simulink model "rev_3f_UW"  (Simulink 8.4)
settings: Solver=ode23tb  StartTime=0.0  StopTime=0.3  MaxStep=2e-4  RelTol=1e-3  AbsTol=1e-6
libraries: powerlib x22, powerlib_extras x6
settings Model: Creator=Teacher  LastModifiedBy=Student
settings SolverCC: ZeroCrossAlgorithm=Adaptive
settings DataIOCC: LimitDataPoints=off  SaveOutput=off  SaveTime=off
settings OptimizationCC: BlockReduction=off  BooleanDataType=off  ExpressionDepthLimit=128  InitFltsAndDblsToZero=on
settings DebuggingCC: SaveWithParameterizedLinksMsg=none  SignalResolutionControl=TryResolveAllWithWarning  SolverPrmCheckMsg=none  MultiTaskDSMMsg=warning  MultiTaskCondExecSysMsg=none  StateNameClashWarn=none
settings HardwareCC: TargetHWDeviceType=32-bit Generic
settings RTWCC: IncludeERTFirstTime=on
settings GRTTargetCC: TargetFcnLib=ansi_tfl_tmw.mat

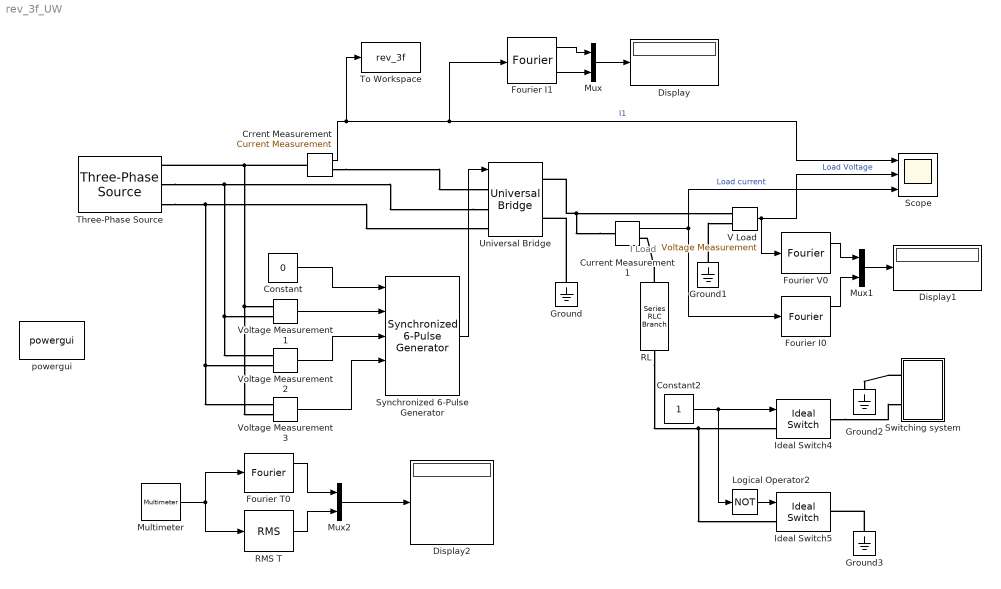
== system rev_3f_UW ==
  note: I Load
  Constant : Constant  Value=0  VectorParams1D=off
  Constant2 : Constant  OutDataTypeStr=boolean
  Crrent Measurement : powerlib/Measurements/Current Measurement  Tag=PoWeRsYsTeMmEaSuReMeNt  PhasorSimulation=off  OutputType=Complex  PSBequivalent=0
  Current Measurement1 : powerlib/Measurements/Current Measurement  PhasorSimulation=off  OutputType=Complex  PSBequivalent=0
  Display : Display
      settings: SampleTime=2e-4
  Display1 : Display
      settings: SampleTime=2e-4
  Display2 : Display
      settings: SampleTime=2e-4
  Fourier I0 : powerlib_extras/Measurements/Fourier  f1=300  n=0
  Fourier I1 : powerlib_extras/Measurements/Fourier  f1=50  n=1
  Fourier T0 : powerlib_extras/Measurements/Fourier  f1=50  n=0
  Fourier V0 : powerlib_extras/Measurements/Fourier  f1=300  n=0
  Ground{,1..3} (4 alike) : powerlib/Elements/Ground  LConnTagsString=a
  Ideal Switch4 : powerlib/Power Electronics/Ideal Switch  Ron=0.1  Lon=0  IC=0  Rs=1e6  Cs=1e-9  Measurements=off
  Ideal Switch5 : powerlib/Power Electronics/Ideal Switch  Ron=0.1  Lon=0  IC=0  Rs=1e6  Cs=1e-9  Measurements=off
  Logical Operator2 : Logic  Operator=NOT  AllPortsSameDT=off  OutDataTypeStr=boolean
  Multimeter : powerlib/Measurements/Multimeter  PhasorSimulation=off  OutputType=Complex  sel=[12 1]  L=17  Gain=[1 1]  yselected={'Isw1: Universal Bridge','Usw1: Universal Bridge'};  PSBOutputType=1  PSBequivalent=0  AxesSetting=[0,0.1,-100,100]  Display=1  SavedBlockNames=-11
  Mux : Mux  Inputs=2
  Mux1 : Mux  Inputs=2
  Mux2 : Mux  Inputs=2
  RL : powerlib/Elements/Series RLC Branch  LConnTagsString=__new0  RConnTagsString=__new0  BranchType=RL  Resistance=10  Inductance=10*10/(2*pi*300)  SetiL0=off  InitialCurrent=0  Capacitance=inf  Setx0=off  InitialVoltage=0  Measurements=None
  RMS T : powerlib_extras/Measurements/RMS  f1=50
  Scope : Scope  NumInputPorts=3
      settings: TimeRange=1  YMin=-15~-500~0  YMax=15~600~13
  Switching system : Subsystem
  Synchronized 6-Pulse Generator : powerlib_extras/Control  Blocks/Synchronized 6-Pulse Generator  freq=50  pwidth=10  Double_Pulse=off
  Three-Phase Source : powerlib/Electrical Sources/Three-Phase Source  Voltage=560*sqrt(1.5)  PhaseAngle=0  Frequency=50  InternalConnection=Yn  SpecifyImpedance=off  Resistance=0.005  Inductance=0  ShortCircuitLevel=100e6  BaseVoltage=560*sqrt(1.5)  XRratio=7  BusType=swing  Pref=0  Qref=0  Qmin=-inf  Qmax=inf
  To Workspace : ToWorkspace  VariableName=rev_3f  SampleTime=2e-4
      settings: MaxDataPoints=200
  Universal Bridge : powerlib/Power Electronics/Universal Bridge  Arms=3  SnubberResistance=1e6  SnubberCapacitance=1e-9  Device=Thyristors  Ron=0.1  Lon=0  ForwardVoltages="[  0  0  ]"  ForwardVoltage=2  GTOparameters=[ 10e-6 , 20e-6 ]  IGBTparameters=[ 1e-6 , 2e-6 ]  Measurements=All voltages and currents  Measurements_2=None  converterType=Rectifier
  V Load : powerlib/Measurements/Voltage Measurement  PhasorSimulation=off  OutputType=Complex  PSBequivalent=0
  Voltage Measurement1 : powerlib/Measurements/Voltage Measurement  PhasorSimulation=off  OutputType=Complex  PSBequivalent=0
  Voltage Measurement2 : powerlib/Measurements/Voltage Measurement  PhasorSimulation=off  OutputType=Complex  PSBequivalent=0
  Voltage Measurement3 : powerlib/Measurements/Voltage Measurement  PhasorSimulation=off  OutputType=Complex  PSBequivalent=0
  powergui : powerlib/powergui  Priority=1  SimulationMode=Discrete  SolverType=Tustin/Backward Euler (TBE)  SampleTime=2e-4  frequency=60  SPID=off  DisableSnubberDevices=off  DisableRonSwitches=off  DisableVfSwitches=off  SwTol=0  DisplayEquations=off  Interpol=off  methode=off  Ts=100  frequencyindice=50  Pbase=100e6  ErrMax=1e-4  Iterations=50  UnitsV=kV  UnitsW=MW  FunctionMessages=off  echomessages=off  HookPort=off  EnableUseOfTLC=off  x0status=blocks  RestoreLinks=warning  ResistiveCurrentMeasurement=off  Frange=[0:2:500]  Ylog=off  Xlog=on  ShowGrid=off  save=off  variable=ZData  structure=0  ZoomFFT=off  StartTime=0.0  cycles=1  DisplayStyle=1  fundamental=60  FreqAxis=off  MaxFrequency=1000  frequencyindicesteady=1  RmsSteady=1  display=off
  wires:
  Fourier I1/1 -> Mux/1
  Fourier I1/2 -> Mux/2
  Fourier I0/1 -> Mux1/2
  Fourier V0/1 -> Mux1/1
  V Load/1 -> Fourier V0/1, Scope/2  "Load Voltage"
  Current Measurement1/1 -> Fourier I0/1, Scope/3  "Load current"
  Mux1/1 -> Display1/1
  Mux/1 -> Display/1
  Voltage Measurement1/1 -> Synchronized 6-Pulse Generator/2
  Voltage Measurement2/1 -> Synchronized 6-Pulse Generator/3
  Voltage Measurement3/1 -> Synchronized 6-Pulse Generator/4
  Constant/1 -> Synchronized 6-Pulse Generator/1
  Synchronized 6-Pulse Generator/1 -> Universal Bridge/1
  Crrent Measurement/1 -> Fourier I1/1, Scope/1, To Workspace/1  "I1"
  Constant2/1 -> Ideal Switch4/1, Logical Operator2/1
  Logical Operator2/1 -> Ideal Switch5/1
  Multimeter/1 -> Fourier T0/1, RMS T/1
  Mux2/1 -> Display2/1
  Fourier T0/1 -> Mux2/1
  RMS T/1 -> Mux2/2
  connections:
  Crrent Measurement/RConn1 -- Universal Bridge/LConn1
  Current Measurement1/LConn1 -- Universal Bridge/RConn1 -- V Load/LConn1
  RL/LConn1 -- Current Measurement1/RConn1
  Ground/LConn1 -- Universal Bridge/RConn2
  Ground1/LConn1 -- V Load/LConn2
  Crrent Measurement/LConn1 -- Three-Phase Source/RConn1 -- Voltage Measurement3/LConn2 -- Voltage Measurement1/LConn1
  Universal Bridge/LConn2 -- Three-Phase Source/RConn2 -- Voltage Measurement2/LConn1 -- Voltage Measurement1/LConn2
  Three-Phase Source/RConn3 -- Universal Bridge/LConn3 -- Voltage Measurement3/LConn1 -- Voltage Measurement2/LConn2
  RL/RConn1 -- Ideal Switch4/LConn1 -- Ideal Switch5/LConn1
  Ground3/LConn1 -- Ideal Switch5/RConn1
  Switching system/LConn1 -- Ground2/LConn1
  Ideal Switch4/RConn1 -- Switching system/LConn2

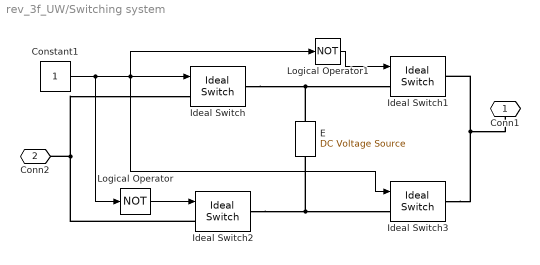
== system rev_3f_UW/Switching system ==
  Constant1 : Constant  OutDataTypeStr=boolean
  E : powerlib/Electrical Sources/DC Voltage Source  Amplitude=100  Measurements=Voltage
  Ideal Switch{,1..3} (4 alike) : powerlib/Power Electronics/Ideal Switch  Ron=0.1  Lon=0  IC=0  Rs=1e6  Cs=1e-9  Measurements=off
  Logical Operator : Logic  Operator=NOT  AllPortsSameDT=off  OutDataTypeStr=boolean
  Logical Operator1 : Logic  Operator=NOT  AllPortsSameDT=off  OutDataTypeStr=boolean
  Conn1 : PMIOPort  Port=1  Side=Left
  Conn2 : PMIOPort  Port=2  Side=Left
  wires:
  Constant1/1 -> Ideal Switch/1, Ideal Switch3/1, Logical Operator1/1, Logical Operator/1
  Logical Operator/1 -> Ideal Switch2/1
  Logical Operator1/1 -> Ideal Switch1/1
  connections:
  E/LConn1 -- Ideal Switch2/RConn1 -- Ideal Switch3/LConn1
  E/RConn1 -- Ideal Switch/RConn1 -- Ideal Switch1/LConn1
  Conn2/RConn1 -- Ideal Switch2/LConn1 -- Ideal Switch/LConn1
  Conn1/RConn1 -- Ideal Switch3/RConn1 -- Ideal Switch1/RConn1
